simulink model "SF5_5_8_na001"  (R2016b)
settings: Solver=VariableStepAuto  StartTime=0.0  StopTime=10.0  RelTol=1e-3
settings Model: Creator=amyyang  LastModifiedBy=amyyang

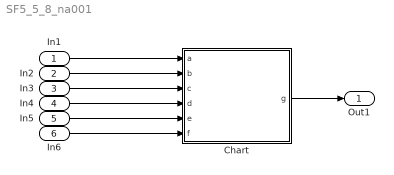
== system SF5_5_8_na001 ==
  In1 : Inport
  In2 : Inport  Port=2
  In3 : Inport  Port=3
  In4 : Inport  Port=4
  In5 : Inport  Port=5
  In6 : Inport  Port=6
  Chart : Stateflow chart  TreatAsAtomicUnit=on
  Out1 : Outport
  wires:
  In1/1 -> Chart/1(a)
  In2/1 -> Chart/2(b)
  In3/1 -> Chart/3(c)
  In4/1 -> Chart/4(d)
  In5/1 -> Chart/5(e)
  In6/1 -> Chart/6(f)
  Chart/1(g) -> Out1/1

== stateflow chart SF5_5_8_na001/Chart ==
  note: 布尔数据类型逻辑操作
  note: 整型的位运算
  (default) -> (junction 2)
  (junction 2) -> (junction 6) [order 1] : [ (a||b)&&c]
  (junction 2) -> (junction 3) [order 2]
  (junction 6) -> (junction 5) : {
      |  g = (d|e)&f;
      | }
  (junction 5) -> (junction 3)
  (junction 3) -> (junction 10)
  data: a input boolean; b input boolean; c input boolean; d input uint8; e input uint8; f input uint8; g output uint8
